simulink model "Suspension_System_in_automobile"  (R2021a)
settings: Solver=VariableStepAuto  StartTime=0.0  StopTime=50  RelTol=1e-3
model workspace (MAT data in the model file):
  b1 = 350
  b2 = 15020
  k1 = 80000
  k2 = 500000
  m1 = 2500
  m2 = 320
settings Model: Creator=91839  LastModifiedBy=91839

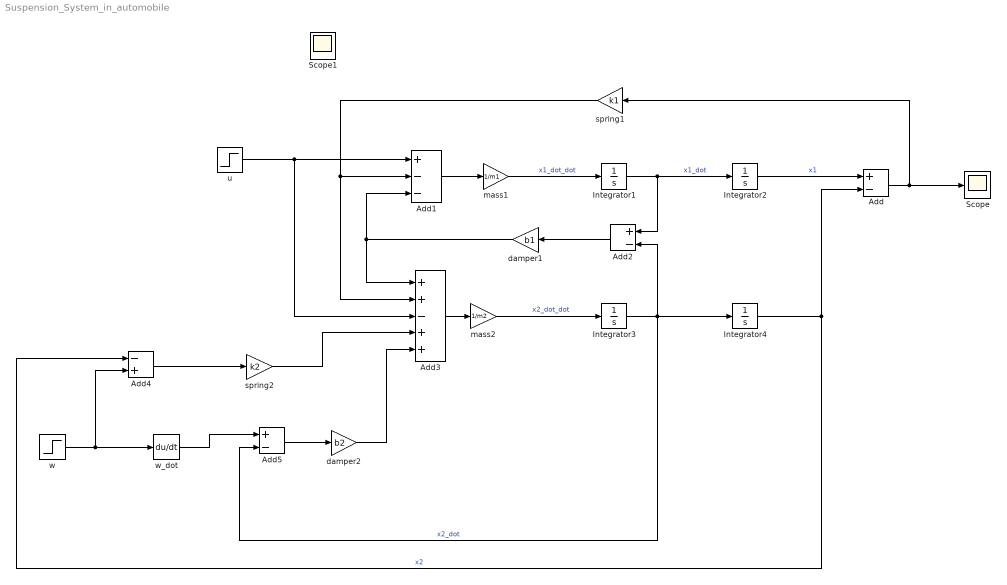
== system Suspension_System_in_automobile ==
  Add : Sum  Inputs=+-
  Add1 : Sum  Inputs=+--
  Add2 : Sum  Inputs=+-
  Add3 : Sum  Inputs=++-++
  Add4 : Sum  Inputs=-+
  Add5 : Sum  Inputs=+-
  Integrator{1..4} (4 alike) : Integrator
  Scope : Scope
  damper1 : Gain  Gain=b1
  damper2 : Gain  Gain=b2
  mass1 : Gain  Gain=1/m1
  mass2 : Gain  Gain=1/m2
  spring1 : Gain  Gain=k1
  spring2 : Gain  Gain=k2
  u : Step  Time=0  SampleTime=0
  w : Step  Time=0  SampleTime=0
  w_dot : Derivative
  Scope1 : Scope
  wires:
  mass1/1 -> Integrator1/1  "x1_dot_dot"
  Integrator1/1 -> Add2/1, Integrator2/1  "x1_dot"
  Integrator2/1 -> Add/1  "x1"
  mass2/1 -> Integrator3/1  "x2_dot_dot"
  Integrator3/1 -> Add5/2, Add2/2, Integrator4/1  "x2_dot"
  Integrator4/1 -> Add4/1, Add/2  "x2"
  Add/1 -> Scope/1, spring1/1
  Add1/1 -> mass1/1
  spring1/1 -> Add3/2, Add1/2
  Add2/1 -> damper1/1
  damper1/1 -> Add1/3, Add3/1
  Add3/1 -> mass2/1
  w/1 -> w_dot/1, Add4/2
  Add4/1 -> spring2/1
  Add5/1 -> damper2/1
  u/1 -> Add3/3, Add1/1
  spring2/1 -> Add3/4
  damper2/1 -> Add3/5
  w_dot/1 -> Add5/1
